simulink model "Cv_7_simulink_model"  (R2024a)
settings: Solver=FixedStepAuto  StartTime=0.0  StopTime=500  FixedStep=1e-3  MaxStep=1e-3  RelTol=1e-3
InitFcn:
  | Cv_7_init
values from neighbouring files (symbols this model uses):
  b = 2    [Cv_7_init.m]
  F0 = 1    [Cv_7_init.m]
  k = 50    [Cv_7_init.m]
  m = 1    [Cv_7_init.m]
  omega = 5    [Cv_7_init.m]
  v_0 = 0    [Cv_7_init.m]
  x_0 = 0    [Cv_7_init.m]
libraries: simulink x1
settings Model: Creator=221208  LastModifiedBy=Miloš Uhlíř
settings ModelReferenceCC: EnableRefExpFcnMdlSchedulingChecks=on
settings RTWCC: GPUComputeCapability=3.5

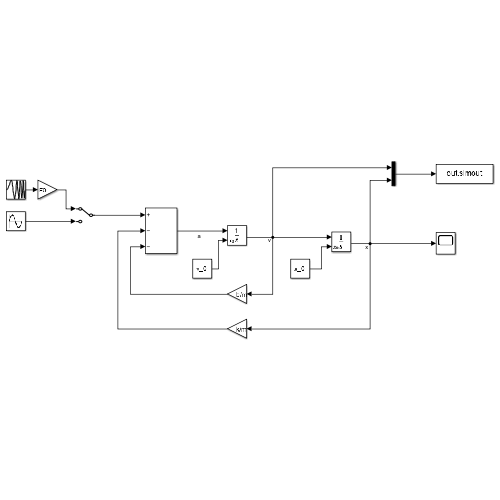
[thumbnail: Simulink's stored preview of the top-level diagram]
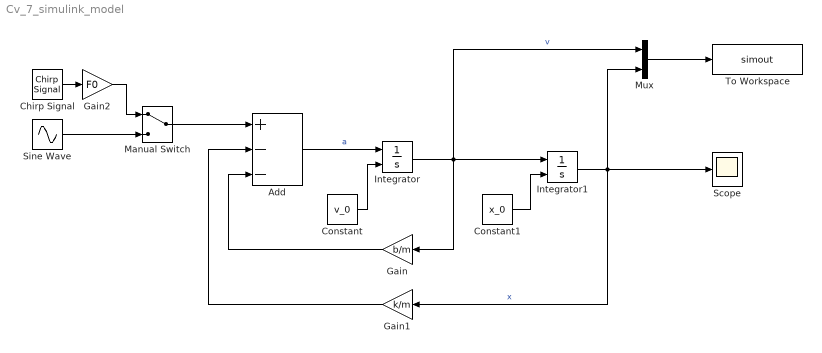
== system Cv_7_simulink_model ==
  Add : Sum  Inputs=+--
  Chirp Signal : simulink/Sources/Chirp Signal  f1=0  T=500  f2=5
  Constant : Constant  Value=v_0
  Constant1 : Constant  Value=x_0
  Gain : Gain  Gain=b/m
  Gain1 : Gain  Gain=k/m
  Gain2 : Gain  Gain=F0
  Integrator : Integrator  InitialConditionSource=external
  Integrator1 : Integrator  InitialConditionSource=external
  Manual Switch : ManualSwitch
  Mux : Mux  Inputs=2
  Scope : Scope
  Sine Wave : Sin  Amplitude=F0  Frequency=omega  SampleTime=0
  To Workspace : ToWorkspace  VariableName=simout  SaveFormat=Timeseries  SampleTime=-1
  wires:
  Add/1 -> Integrator/1  "a"
  Integrator/1 -> Gain/1, Mux/1, Integrator1/1  "v"
  Integrator1/1 -> Gain1/1, Scope/1, Mux/2  "x"
  Gain/1 -> Add/3
  Gain1/1 -> Add/2
  Mux/1 -> To Workspace/1
  Constant1/1 -> Integrator1/2
  Constant/1 -> Integrator/2
  Sine Wave/1 -> Manual Switch/2
  Manual Switch/1 -> Add/1
  Chirp Signal/1 -> Gain2/1
  Gain2/1 -> Manual Switch/1
